simulink library "RouterBtc"  (R2022b)
settings: Solver=VariableStepAuto  StartTime=0.0  StopTime=10.0  RelTol=1e-3
undefined symbols (not defined in the file or in its folder): Column
libraries: TuneVar x2, simulink x2, FeaturePath x1, HandyTextFile x1, RTC x1, TOP x1, dspindex x1
settings Model: Creator=kl13806  LastModifiedBy=kl13806
settings SolverCC: AlgebraicLoopSolver=TrustRegion
settings DebuggingCC: UnconnectedInputMsg=warning  UnconnectedOutputMsg=warning  UnconnectedLineMsg=warning  SFMachineParentedDataDiag=warning
settings ModelReferenceCC: EnableRefExpFcnMdlSchedulingChecks=on
settings RTWCC: DLArmComputeVersion=19.05

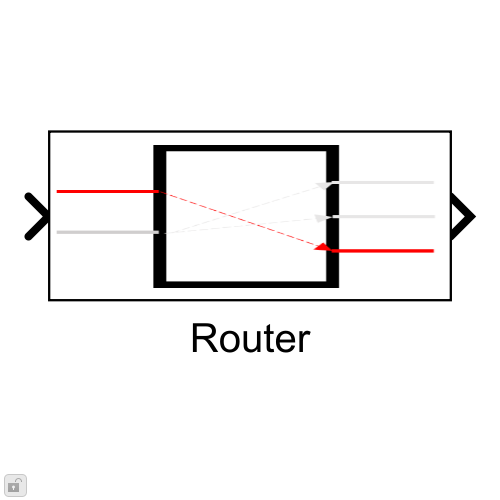
[thumbnail: Simulink's stored preview of the top-level diagram]
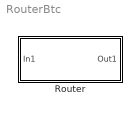
== system RouterBtc ==
  Router : Subsystem  mask(Blocklib Router){Config=[], FeatureName=Router}
      mask prompts: Config "RouterConfig"; FeatureName "Feature path name:"
      mask help: This block allows the user to route X input channels to Y output channels. Enter a value of 0 to "zero out" the specific channel
      mask init:
      | blkh=gcbh;
      | Config=BTConfig.Assert(blkh,Config);
      | 
      | Config.Validate();
      | BTConfig.InitSetFeatureIfPresent(blkh,'FeatureName');
      mask Callback Config: BTConfig.CallbackHideIfPresent(gcbh,{'FeatureName'});
      mask TypeOptions FeatureName: FeaturePath/FeatureName
      mask Display: image('routerIcon.png');

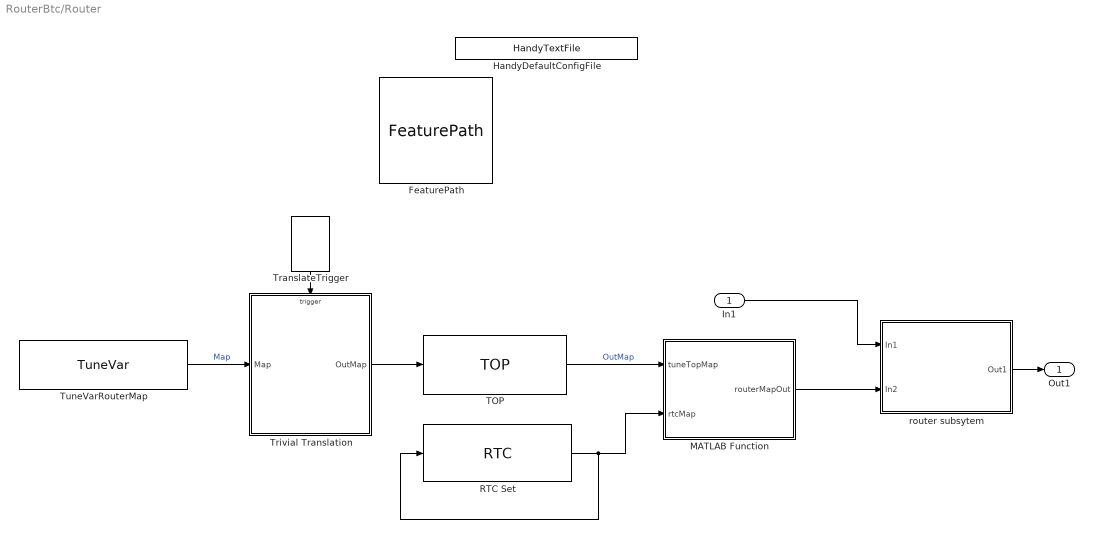
== system RouterBtc/Router ==
  In1 : Inport
  FeaturePath : FeaturePath/FeaturePath  FeatureName=Router  IsGroup=off  GroupNumber=-1  IsModule=off  TriggerInit=[615 164 730 271]
      settings: SourceProductName=Bose Talaria
  HandyDefaultConfigFile : HandyTextFile/HandyTextFile  TemplateSource=Config  FileSuffix=Init  OpenDialogOnLoad=off  UseThisBlockName=off  AddGrandParentNamePrefix=off  TheDefaultText=|  ShowInLibBrowser=on
      | % $(FILENAME) Setup model parameters for each "Init" callback (e.g. update diagram)
      | sample_rate_in_hertz = 44100;
      | frame_size = 32;
      | sysin_channel_count = 2;
      settings: SourceProductName=Bose Talaria
  MATLAB Function : MATLAB Function  TreatAsAtomicUnit=on
  RTC Set : RTC/RTC  REQ_Priority=RTC_Mask.NormalPriority  RequestAtInit=off  EnableRequest=off  REQElemName1=routerMap  REQElemType1=int32  REQElemWidth1=Config.NumOut  REQElemInitial1=[]  REQElemType2=uint32  REQElemWidth2=1  REQElemInitial2=[]  REQElemType3=uint32  REQElemWidth3=1  REQElemInitial3=[]  REQElemType4=uint32  REQElemWidth4=1  REQElemInitial4=[]  REQElemType5=uint32  REQElemWidth5=1  REQElemInitial5=[]  REQElemType6=uint32  REQElemWidth6=1  REQElemInitial6=[]  REQElemType7=uint32  REQElemWidth7=1  REQElemInitial7=[]  REQElemType8=uint32  REQElemWidth8=1  REQElemInitial8=[]  REQElemType9=uint32  REQElemWidth9=1  REQElemInitial9=[]  REQElemType10=uint32  REQElemWidth10=1  REQElemInitial10=[]  EnableResponse=on  EnableRSP_StatusIn=off  RSPElemName1=routerMap  RSPElemType1=int8  RSPElemWidth1=Config.NumOut  RSPElemType2=uint32  RSPElemWidth2=1  RSPElemType3=uint32  RSPElemWidth3=1  RSPElemType4=uint32  RSPElemWidth4=1  RSPElemType5=uint32  RSPElemWidth5=1  RSPElemType6=uint32  RSPElemWidth6=1  RSPElemType7=uint32  RSPElemWidth7=1  RSPElemType8=uint32  RSPElemWidth8=1  RSPElemType9=uint32  RSPElemWidth9=1  RSPElemType10=uint32  RSPElemWidth10=1  EnableNotification=off  EnableNTF_PrepTrig=off  NTFElemType1=uint32  NTFElemWidth1=1  NTFElemType2=uint32  NTFElemWidth2=1  NTFElemType3=uint32  NTFElemWidth3=1  NTFElemType4=uint32  NTFElemWidth4=1  NTFElemType5=uint32  NTFElemWidth5=1  NTFElemType6=uint32  NTFElemWidth6=1  NTFElemType7=uint32  NTFElemWidth7=1  NTFElemType8=uint32  NTFElemWidth8=1  NTFElemType9=uint32  NTFElemWidth9=1  NTFElemType10=uint32  NTFElemWidth10=1  MaskMessageName=Set
      settings: SourceProductName=Bose Talaria
  TOP : TOP/TOP  TriggerInit=[660 425 805 485]  TopName=OutMap  DataType=int32  BankNumber=0  PreOverlay=false  PostOverlay=false  Role=Automatic
      settings: SourceProductName=Bose Talaria
  TranslateTrigger : TuneVar/TranslateTrigger  TriggerInit=[526 305 564 360]
      settings: SourceProductName=Bose Talaria
  Trivial Translation : MATLAB Function  TreatAsAtomicUnit=on  mask{nInRouterMask=Config.NumIn}
      mask prompts: nInRouterMask "Num Input"
  TuneVarRouterMap : TuneVar/TuneVar  TuneName=Map  SpecifyMaxSize=on  VariableDim=2 (Column)  MaxSize=[1 Config.NumOut]  TunabilityNumber=1  MinValue=[]  MaxValue=[]  TriggerInit=[250 430 420 480]  MaskValue=Config.DefaultOutputMap
      settings: SourceProductName=Bose Talaria
  router subsytem : Subsystem
  Out1 : Outport  VectorParamsAs1DForOutWhenUnconnected=off
  wires:
  router subsytem/1(Out1) -> Out1/1
  TOP/1 -> MATLAB Function/1(tuneTopMap)  "OutMap"
  TuneVarRouterMap/1 -> Trivial Translation/1(Map)  "Map"
  Trivial Translation/1(OutMap) -> TOP/1
  In1/1 -> router subsytem/1(In1)
  TranslateTrigger/1 -> Trivial Translation/Trigger
  RTC Set/1 -> MATLAB Function/2(rtcMap), RTC Set/1
  MATLAB Function/1(routerMapOut) -> router subsytem/2(In2)

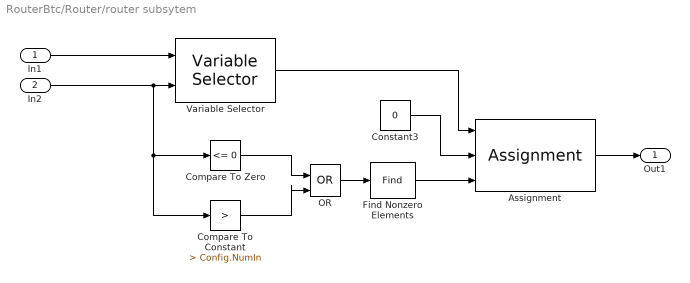
== system RouterBtc/Router/router subsytem ==
  In1 : Inport
  In2 : Inport  Port=2
  Assignment : Assignment  NumberOfDimensions=2  DiagnosticForDimensions=Warning  IndexOptions=Assign all,Index vector (port)  Indices=1,[1 3]  OutputSizes=1,1
  Compare To Constant : simulink/Logic and Bit Operations/Compare To Constant  relop=>  const=Config.NumIn  OutDataTypeStr=boolean
  Compare To Zero : simulink/Logic and Bit Operations/Compare To Zero  relop=<=  OutDataTypeStr=boolean
  Constant3 : Constant  Value=0  OutDataTypeStr=single
  Find Nonzero Elements : Find  NumberOfInputDimensions=3
  OR : Logic  Operator=OR  IconShape=distinctive  AllPortsSameDT=off  OutDataTypeStr=boolean
  Variable Selector : dspindex/Variable Selector  NumInputs=1  rowsOrCols=Columns  IdxMode=Variable  Elements=[3]  ZerOneIdxMode=One-based  errmode=Clip Index  FillMode=on  FillValues=0
  Out1 : Outport  VectorParamsAs1DForOutWhenUnconnected=off
  wires:
  Compare To Constant/1 -> OR/2
  Assignment/1 -> Out1/1
  OR/1 -> Find Nonzero Elements/1
  In2/1 -> Variable Selector/2, Compare To Zero/1, Compare To Constant/1
  Variable Selector/1 -> Assignment/1
  Find Nonzero Elements/1 -> Assignment/3
  In1/1 -> Variable Selector/1
  Compare To Zero/1 -> OR/1
  Constant3/1 -> Assignment/2

== matlab function RouterBtc/Router/Trivial Translation ==
  data: OutMap output; Map input; nInRouterMask parameter
  events: trigger input FUNCTION_CALL_EVENT
function OutMap  = fcn(Map, nInRouterMask)
%#codegen

% ----- To access TuneVar maximum size, current size, and current value:
%   Note: TuneVar signals arrive with exposed variable size information.
%         The expressions below illustrate for the "Map" input argument.
%
%   size(Map.Value) : the maximum possible size of the Map variable
%
%   Tune.Size   : the current size of *valid* data in Map.Value
%
%   Map.Size(1) : Number of rows present in Map - this does not vary.
%
%   Map.Size(2) : Number of columns currently valid in Map - this is
%       the variable part of size that can change (if allowed by TuneVar).
%
%   Map.Value : the current value of the tune variable... but end-padded 
%       to the maximum available size with undefined/invalid data.
%
%   numel(Map.Value) : another way of looking at the maximum number of
%       elements that could arrive in Map.Value
%
% ----- To register an error, use the following method (works like printf):
%   TranslateError( <format string>, <arguments ... )
%   ... this error will cause the build process to abort.


% The below logic ensures that an output map gets filled in in the 
% "round robin" manner. This is to occur when the supplied map is shorter
% than the number of channel outputs. For instance,
% nChanIn = 4
% nChanOut = 9
% outputMapSupplied = [4 3 2 2]
% 
% This logic would run and return OutMap = [4 3 2 2 1 2 3 4 1]
%
% If no outputMap was supplied (i.e. = [];) THEN
% This logic would run and return OutMap = [1 2 3 4 1 2 3 4 1];


% First part finds the number of output map indices that were left blank
nChanOut = numel(Map.Value);
mapLength = Map.Size(2);
mapDifference = nChanOut - mapLength;
OutMap = int32(Map.Value);

% This loop appropriates the correct input channel number to the
% corresponding output channel, based on the mapDifference found above
if (mapLength == 1) && Map.Value(1) == 0
    mapLength = 0;
    mapDifference = nChanOut;
end
endOfMap = 0;
loopCount = 0;
while endOfMap < mapDifference
    for inputChan = 1 : nInRouterMask
        OutMap(mapLength+inputChan+loopCount) = inputChan;
        endOfMap = endOfMap + 1;
        if endOfMap == mapDifference
            break
        end
    end
    inputChan = 1;
    loopCount = loopCount + nInRouterMask;
end

== matlab function RouterBtc/Router/MATLAB Function ==
  data: tuneTopMap input; routerMapOut output; rtcMap input
function routerMapOut = choose_correct_map(tuneTopMap, rtcMap)

% tuneTopMap is provided via a tune variable. However 
% if parameters are provided through RTC, the block will use the values 
% given in the RTC messages.

Numiters=size(rtcMap,1);
routerMapOut = int32(tuneTopMap);
for ind=1:Numiters
    if (rtcMap(ind))
        routerMapOut(ind) = rtcMap(ind);        
    end
end
